simulink model "simulinkCollision"  (R2017a)
settings: Solver=VariableStepAuto  StartTime=0.0  StopTime=10.0  RelTol=1e-3
PreLoadFcn:
  | % Body 1 properties
  | m1 = 1;
  | v1 = 1;
  | x1 = 0;
  | 
  | % Body 2 properties
  | m2 = 5;
  | v2 = -0.1;
  | x2 = 5;
  | 
  | % Coefficient of restitution
  | % 0 = inelastic, 1 = elastic
  | Cr = 0.5;
libraries: simulink x1
settings Model: Creator=scastro  LastModifiedBy=scastro

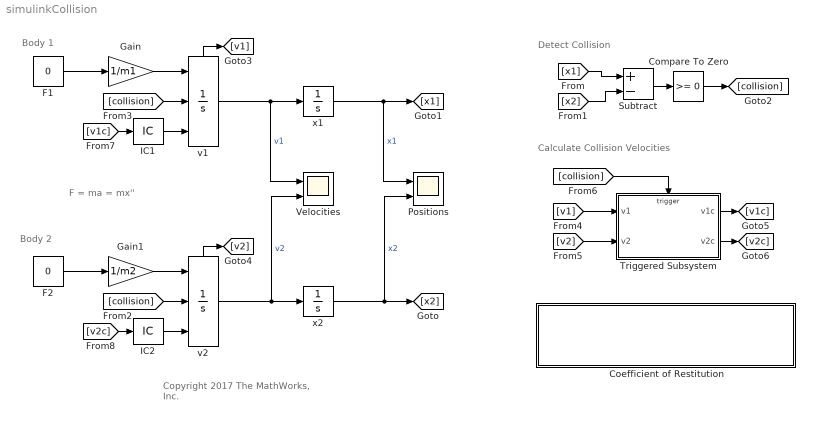
== system simulinkCollision ==
  note: F = ma = mx''
  note: Body 1
  note: Body 2
  note: Calculate Collision Velocities
  note: Detect Collision
  note: Copyright 2017 The MathWorks, Inc.
  Coefficient of Restitution : Subsystem  DialogController=hmiCreateDDGDialog  IsWebBlock=on  mask(MWDashboardBlock){webBlockId=c01f5e7b-c93b-41b5-9ddf-3a19c4bf8f87, webBlockType=slider, ShowInLibBrowser=on, ShowInitialText=on, HMISrcModelName=simulinkCollision}
      mask prompts: webBlockId "WebBlock Id"; webBlockType "WebBlock Type"; HMISrcModelName "Source Model"
      mask help: SimulinkHMI:dialogs:SliderDialogDesc
      mask Help: helpview([docroot '/mapfiles/simulink.map'], 'hmi_slider')
      mask Display:
      | if strcmp(get_param(bdroot(gcb),'BlockDiagramType'), 'library')
      |     image([(matlabroot) '/toolbox/simulink/hmi/icons/Slider.png']);
      | end
  Compare To Zero : simulink/Logic and Bit Operations/Compare To Zero  relop=>=  OutDataTypeStr=boolean
  F1 : Constant  Value=0
  F2 : Constant  Value=0
  Gain : Gain  Gain=1/m1
  Gain1 : Gain  Gain=1/m2
  IC1 : InitialCondition  Value=v1
  IC2 : InitialCondition  Value=v2
  Positions : Scope  NumInputPorts=2
  Subtract : Sum  Inputs=+-
  Triggered Subsystem : Subsystem  TreatAsAtomicUnit=on
  Velocities : Scope  NumInputPorts=2
  v1 : Integrator  ExternalReset=rising  InitialConditionSource=external  InitialCondition=v1  ShowStatePort=on
  v2 : Integrator  ExternalReset=rising  InitialConditionSource=external  InitialCondition=v2  ShowStatePort=on
  x1 : Integrator  InitialCondition=x1
  x2 : Integrator  InitialCondition=x2
  wires:
  v1/1 -> Velocities/1, x1/1  "v1"
  F1/1 -> Gain/1
  Gain/1 -> v1/1
  Gain1/1 -> v2/1
  F2/1 -> Gain1/1
  v2/1 -> x2/1, Velocities/2  "v2"
  Subtract/1 -> Compare To Zero/1
  [x1] -> Subtract/1
  [x2] -> Subtract/2
  Compare To Zero/1 -> [collision]
  [collision] -> v2/2
  [collision] -> v1/2
  x1/1 -> Positions/1, [x1]  "x1"
  x2/1 -> Positions/2, [x2]  "x2"
  v1/State -> [v1]
  v2/State -> [v2]
  [v1] -> Triggered Subsystem/1(v1)
  [v2] -> Triggered Subsystem/2(v2)
  [collision] -> Triggered Subsystem/Trigger
  Triggered Subsystem/1(v1c) -> [v1c]
  Triggered Subsystem/2(v2c) -> [v2c]
  [v1c] -> IC1/1
  [v2c] -> IC2/1
  IC1/1 -> v1/3
  IC2/1 -> v2/3

== system simulinkCollision/Coefficient of Restitution ==

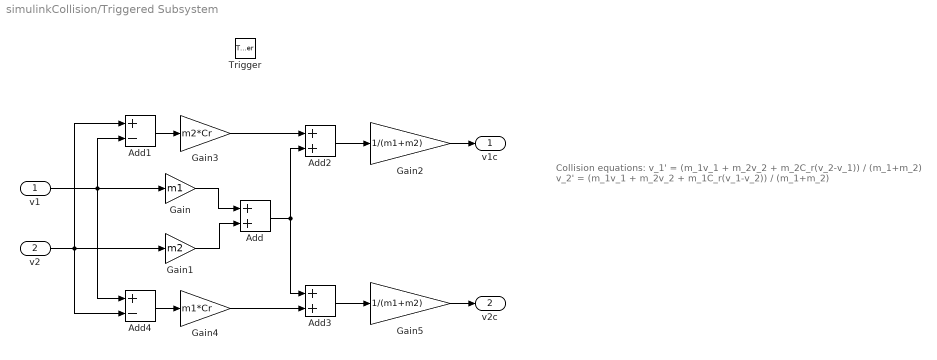
== system simulinkCollision/Triggered Subsystem ==
  note: Collision equations:
      |
      | v_1' = (m_1v_1 + m_2v_2 + m_2C_r(v_2-v_1)) / (m_1+m_2)
      |
      | v_2' = (m_1v_1 + m_2v_2 + m_1C_r(v_1-v_2)) / (m_1+m_2)
  v1 : Inport
  v2 : Inport  Port=2
  Trigger : TriggerPort  VariantControl=Variant
  Add : Sum
  Add1 : Sum  Inputs=+-
  Add2 : Sum
  Add3 : Sum
  Add4 : Sum  Inputs=+-
  Gain : Gain  Gain=m1
  Gain1 : Gain  Gain=m2
  Gain2 : Gain  Gain=1/(m1+m2)
  Gain3 : Gain  Gain=m2*Cr
  Gain4 : Gain  Gain=m1*Cr
  Gain5 : Gain  Gain=1/(m1+m2)
  v1c : Outport
  v2c : Outport  Port=2
  wires:
  v1/1 -> Add4/1, Gain/1, Add1/2
  v2/1 -> Gain1/1, Add4/2, Add1/1
  Gain/1 -> Add/1
  Gain1/1 -> Add/2
  Add2/1 -> Gain2/1
  Add1/1 -> Gain3/1
  Gain3/1 -> Add2/1
  Add/1 -> Add2/2, Add3/1
  Gain2/1 -> v1c/1
  Add4/1 -> Gain4/1
  Gain4/1 -> Add3/2
  Add3/1 -> Gain5/1
  Gain5/1 -> v2c/1
